simulink model "simulation2"  (R2021a)
settings: Solver=FixedStepAuto  StartTime=0.0  StopTime=10.0  RelTol=1e-3
values from neighbouring files (symbols this model uses):
  g = 9.8    [invertedp.m]
  K = [-35 -34 -150 -34]    [invertedp.m]
undefined symbols (not defined in the file or in its folder): a, F_v, iM_d, iner, iner_l, K_d, K_p, o_r, pi_l, pi_m, q_i, Tc
settings Model: Creator=jonathanbopp  LastModifiedBy=jonathanbopp

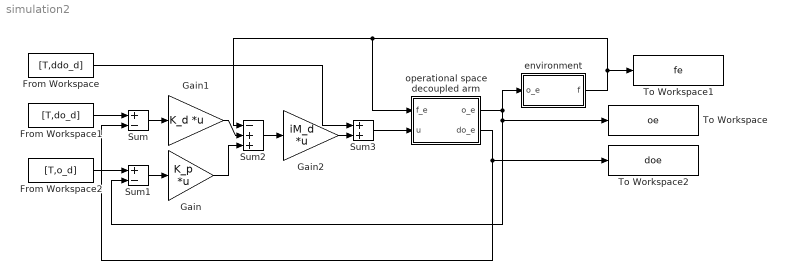
== system simulation2 ==
  From Workspace : FromWorkspace  VariableName=[T,ddo_d]  SampleTime=Tc
  From Workspace1 : FromWorkspace  VariableName=[T,do_d]  SampleTime=Tc
  From Workspace2 : FromWorkspace  VariableName=[T,o_d]  SampleTime=Tc
  Gain : Gain  Gain=K_p  Multiplication=Matrix(K*u)
  Gain1 : Gain  Gain=K_d  Multiplication=Matrix(K*u)
  Gain2 : Gain  Gain=iM_d  Multiplication=Matrix(K*u)
  Sum : Sum  Inputs=+-
  Sum1 : Sum  Inputs=+-
  Sum2 : Sum  Inputs=-||+||+
  Sum3 : Sum
  To Workspace : ToWorkspace  VariableName=oe  SaveFormat=Timeseries  SampleTime=-1
  To Workspace1 : ToWorkspace  VariableName=fe  SaveFormat=Timeseries  SampleTime=-1
  To Workspace2 : ToWorkspace  VariableName=doe  SaveFormat=Timeseries  SampleTime=-1
  environment : Subsystem
      mask Display: disp('K(o_e-o_r)')
  operational space decoupled arm : Subsystem
      mask Display: disp('u = ddo_e')
  wires:
  operational space decoupled arm/1(o_e) -> To Workspace/1, Sum1/2, environment/1(o_e)
  Sum3/1 -> operational space decoupled arm/2(u)
  From Workspace2/1 -> Sum1/1
  Sum1/1 -> Gain/1
  Gain/1 -> Sum2/3
  Gain1/1 -> Sum2/2
  Sum/1 -> Gain1/1
  From Workspace1/1 -> Sum/1
  Sum2/1 -> Gain2/1
  Gain2/1 -> Sum3/2
  From Workspace/1 -> Sum3/1
  environment/1(f) -> To Workspace1/1, operational space decoupled arm/1(f_e), Sum2/1
  operational space decoupled arm/2(do_e) -> To Workspace2/1, Sum/2

== system simulation2/environment ==
  o_e : Inport
  Matrix gain. : StateSpace  A=[]  B=[]  C=[]  D=K  InitialCondition=0  mask(Matrix gain){K=K}
      mask prompts: K "Gain matrix:"
      mask help: Matrix Gain.
      mask Help: Multiplies input vector by entered matrix to produce output vector (y=Au).
      mask Display: disp('K')
  Sum1 : Sum  Inputs=+-  InputSameDT=on  SaturateOnIntegerOverflow=on  OutDataTypeStr=Inherit: Same as first input
  xo : Constant  Value=o_r  SampleTime=-1
  f : Outport  InitialOutput=0
  wires:
  o_e/1 -> Sum1/1
  Matrix gain./1 -> f/1
  Sum1/1 -> Matrix gain./1
  xo/1 -> Sum1/2

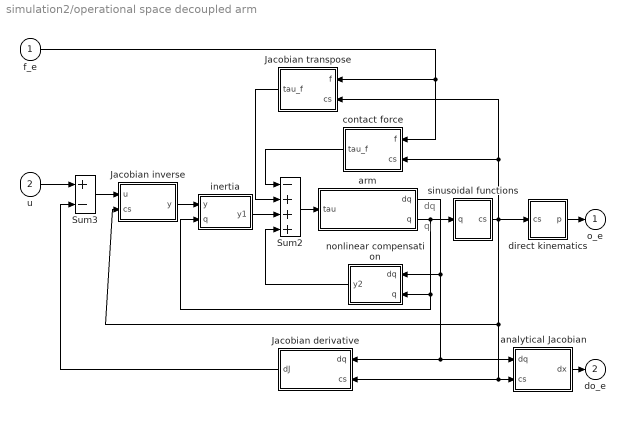
== system simulation2/operational space decoupled arm ==
  note: dq
  note: q
  f_e : Inport
  u : Inport  Port=2
  Jacobian derivative : Subsystem
      mask Display: disp('dJ_a(q,dq)')
  Jacobian inverse : Subsystem
      mask Display: disp('inv(J_a(q))')
  Jacobian transpose : Subsystem
      mask Display: disp('tr(J_a(q))')
  Sum2 : Sum  Inputs=-+++  InputSameDT=on  SaturateOnIntegerOverflow=on  OutDataTypeStr=Inherit: Same as first input
  Sum3 : Sum  Inputs=+-  InputSameDT=on  SaturateOnIntegerOverflow=on  OutDataTypeStr=Inherit: Same as first input
  analytical Jacobian : Subsystem
      mask Display: disp('J_a(q)')
  arm : Subsystem
      mask Display: disp('inv(B(q))(tau-tau'')')
  contact force : Subsystem
      mask Display: disp('tr(J_a(q))f')
  direct kinematics : Subsystem
      mask Display: disp('k(q)')
  inertia : Subsystem
      mask Display: disp('B(q)')
  nonlinear compensation : Subsystem
      mask Display: disp('n(q,dq)')
  sinusoidal functions : Subsystem
      mask Display: disp('cs(q)')
  o_e : Outport  InitialOutput=0
  do_e : Outport  Port=2  InitialOutput=0
  wires:
  f_e/1 -> contact force/1(f), Jacobian transpose/1(f)
  Jacobian transpose/1(tau_f) -> Sum2/2
  inertia/1(y1) -> Sum2/3
  nonlinear compensation/1(y2) -> Sum2/4
  Jacobian derivative/1(dJ) -> Sum3/2
  u/1 -> Sum3/1
  sinusoidal functions/1(cs) -> Jacobian inverse/2(cs), Jacobian derivative/2(cs), analytical Jacobian/2(cs), Jacobian transpose/2(cs), contact force/2(cs), direct kinematics/1(cs)
  contact force/1(tau_f) -> Sum2/1
  arm/2("q ") -> inertia/2(q), nonlinear compensation/2(q), sinusoidal functions/1(q)
  Sum3/1 -> Jacobian inverse/1(u)
  analytical Jacobian/1(dx) -> do_e/1
  direct kinematics/1(p) -> o_e/1
  arm/1(dq) -> nonlinear compensation/1(dq), Jacobian derivative/1(dq), analytical Jacobian/1(dq)
  Sum2/1 -> arm/1(tau)
  Jacobian inverse/1(y) -> inertia/1(y)

== system simulation2/operational space decoupled arm/Jacobian derivative ==
  dq : Inport
  cs : Inport  Port=2
  MATLAB Fcn : MATLABFcn  MATLABFcn=dJ_a  OutputDimensions=2  SampleTime=Tc
      mask Display: disp('dJ_a(q,dq)dq')
  Mux : Mux  Inputs=[2,4]
  dJ : Outport  InitialOutput=0
  wires:
  MATLAB Fcn/1 -> dJ/1
  Mux/1 -> MATLAB Fcn/1
  cs/1 -> Mux/2
  dq/1 -> Mux/1

== system simulation2/operational space decoupled arm/Jacobian inverse ==
  u : Inport
  cs : Inport  Port=2
  MATLAB Fcn : MATLABFcn  MATLABFcn=invJ_a  OutputDimensions=2  SampleTime=Tc
      mask Display: disp('inv(J_a(q))')
  Mux : Mux  Inputs=[2,4]
  y : Outport  InitialOutput=0
  wires:
  u/1 -> Mux/1
  cs/1 -> Mux/2
  Mux/1 -> MATLAB Fcn/1
  MATLAB Fcn/1 -> y/1

== system simulation2/operational space decoupled arm/Jacobian transpose ==
  f : Inport
  cs : Inport  Port=2
  MATLAB Fcn : MATLABFcn  MATLABFcn=trJ_a  OutputDimensions=2  SampleTime=Tc
      mask Display: disp('J''_a(q)f')
  Mux : Mux  Inputs=[2,4]
  tau_f : Outport  InitialOutput=0
  wires:
  cs/1 -> Mux/2
  f/1 -> Mux/1
  Mux/1 -> MATLAB Fcn/1
  MATLAB Fcn/1 -> tau_f/1

== system simulation2/operational space decoupled arm/analytical Jacobian ==
  dq : Inport
  cs : Inport  Port=2
  MATLAB Fcn : MATLABFcn  MATLABFcn=J_adq  OutputDimensions=2
      mask Display: disp('J_a(q)dq')
  Mux : Mux  Inputs=[2,4]
  dx : Outport  InitialOutput=0
  wires:
  cs/1 -> Mux/2
  MATLAB Fcn/1 -> dx/1
  Mux/1 -> MATLAB Fcn/1
  dq/1 -> Mux/1

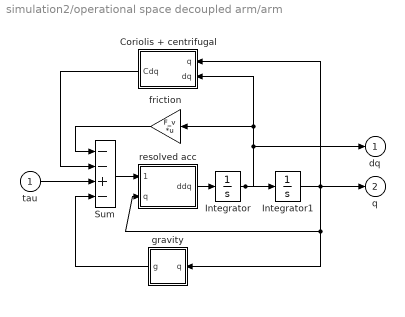
== system simulation2/operational space decoupled arm/arm ==
  tau : Inport
  Coriolis + centrifugal : Subsystem
      mask Display: disp('C(q,dq)dq')
  Integrator : Integrator  InitialCondition=[0 0]  ZeroCross=off
  Integrator1 : Integrator  InitialCondition=q_i  ZeroCross=off
  Sum : Sum  Inputs=--+-  InputSameDT=on  SaturateOnIntegerOverflow=on  OutDataTypeStr=Inherit: Same as first input
  friction : Gain  Gain=F_v  Multiplication=Matrix(K*u)  SaturateOnIntegerOverflow=on  OutDataTypeStr=Inherit: Same as input  ParamDataTypeStr=Inherit: Same as input
      mask Display: disp('F_v')
  gravity : Subsystem
      mask Display: disp('g(q)')
  resolved acc : Subsystem
      mask Display: disp('inv(B(q))')
  dq : Outport  InitialOutput=0
  "q " : Outport  Port=2  InitialOutput=0
  wires:
  gravity/1(g) -> Sum/4
  friction/1 -> Sum/1
  Sum/1 -> resolved acc/1(tau-tau')
  Integrator/1 -> friction/1, Coriolis + centrifugal/2(dq), dq/1, Integrator1/1
  resolved acc/1(ddq) -> Integrator/1
  Integrator1/1 -> "q "/1, gravity/1(q), resolved acc/2(q), Coriolis + centrifugal/1(q)
  tau/1 -> Sum/3
  Coriolis + centrifugal/1(Cdq) -> Sum/2

== system simulation2/operational space decoupled arm/contact force ==
  f : Inport
  cs : Inport  Port=2
  MATLAB Fcn : MATLABFcn  MATLABFcn=trJ_a  OutputDimensions=2
      mask Display: disp('J''_a(q)f')
  Mux : Mux  Inputs=[2,4]
  tau_f : Outport  InitialOutput=0
  wires:
  MATLAB Fcn/1 -> tau_f/1
  Mux/1 -> MATLAB Fcn/1
  cs/1 -> Mux/2
  f/1 -> Mux/1

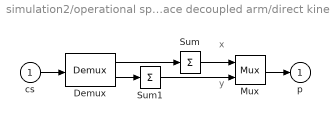
== system simulation2/operational space decoupled arm/direct kinematics ==
  note: y
  note: x
  cs : Inport
  Demux : Demux  Outputs=[2,2]
      settings: DisplayOption=none
  Mux : Mux  Inputs=2
  Sum : Sum  Inputs=+  InputSameDT=on  SaturateOnIntegerOverflow=on  OutDataTypeStr=Inherit: Same as first input
  Sum1 : Sum  Inputs=+  InputSameDT=on  SaturateOnIntegerOverflow=on  OutDataTypeStr=Inherit: Same as first input
  p : Outport  InitialOutput=0
  wires:
  Mux/1 -> p/1
  cs/1 -> Demux/1
  Demux/1 -> Sum/1
  Demux/2 -> Sum1/1
  Sum/1 -> Mux/1
  Sum1/1 -> Mux/2

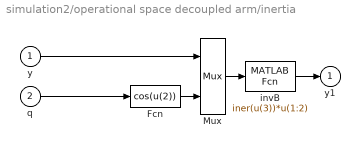
== system simulation2/operational space decoupled arm/inertia ==
  y : Inport
  q : Inport  Port=2
  Fcn : Fcn  Expr=cos(u(2))  SampleTime=Tc
  Mux : Mux  Inputs=[2,1]
  "invB " : MATLABFcn  MATLABFcn=iner(u(3))*u(1:2)  OutputDimensions=2  SampleTime=Tc
      mask Display: disp('B(q)y')
  y1 : Outport  InitialOutput=0
  wires:
  y/1 -> Mux/1
  q/1 -> Fcn/1
  Mux/1 -> "invB "/1
  "invB "/1 -> y1/1
  Fcn/1 -> Mux/2

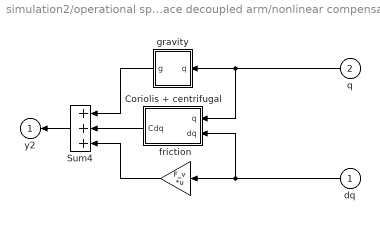
== system simulation2/operational space decoupled arm/nonlinear compensation ==
  dq : Inport
  q : Inport  Port=2
  Coriolis + centrifugal : Subsystem
      mask Display: disp('C(q,dq)dq')
  Sum4 : Sum  Inputs=+++  InputSameDT=on  SaturateOnIntegerOverflow=on  OutDataTypeStr=Inherit: Same as first input
  friction : Gain  Gain=F_v  Multiplication=Matrix(K*u)  SaturateOnIntegerOverflow=on  SampleTime=Tc  OutDataTypeStr=Inherit: Same as input  ParamDataTypeStr=Inherit: Same as input
      mask Display: disp('F_v')
  gravity : Subsystem
      mask Display: disp('g(q)')
  y2 : Outport  InitialOutput=0
  wires:
  Coriolis + centrifugal/1(Cdq) -> Sum4/2
  dq/1 -> friction/1, Coriolis + centrifugal/2(dq)
  q/1 -> Coriolis + centrifugal/1(q), gravity/1(q)
  friction/1 -> Sum4/3
  Sum4/1 -> y2/1
  gravity/1(g) -> Sum4/1

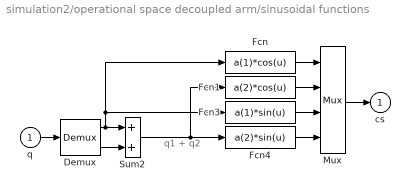
== system simulation2/operational space decoupled arm/sinusoidal functions ==
  note: q1 + q2
  q : Inport
  Demux : Demux  Outputs=2
      settings: DisplayOption=none
  Fcn : Fcn  Expr=a(1)*cos(u)
  Fcn1 : Fcn  Expr=a(2)*cos(u)
  Fcn3 : Fcn  Expr=a(1)*sin(u)
  Fcn4 : Fcn  Expr=a(2)*sin(u)
  Mux : Mux
  Sum2 : Sum  InputSameDT=on  SaturateOnIntegerOverflow=on  OutDataTypeStr=Inherit: Same as first input
  cs : Outport  InitialOutput=0
  wires:
  Fcn/1 -> Mux/1
  Mux/1 -> cs/1
  Demux/1 -> Sum2/1, Fcn3/1, Fcn/1
  Demux/2 -> Sum2/2
  Sum2/1 -> Fcn4/1, Fcn1/1
  Fcn1/1 -> Mux/2
  Fcn3/1 -> Mux/3
  Fcn4/1 -> Mux/4
  q/1 -> Demux/1

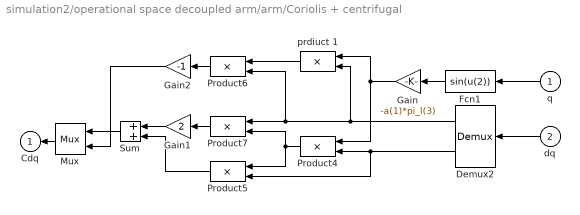
== system simulation2/operational space decoupled arm/arm/Coriolis + centrifugal ==
  q : Inport
  dq : Inport  Port=2
  Demux2 : Demux  Outputs=2
      settings: DisplayOption=none
  Fcn1 : Fcn  Expr=sin(u(2))
  Gain : Gain  Gain=-a(1)*pi_l(3)  SaturateOnIntegerOverflow=on  OutDataTypeStr=Inherit: Same as input  ParamDataTypeStr=Inherit: Same as input
      mask Display: disp('k_3')
  Gain1 : Gain  Gain=2  SaturateOnIntegerOverflow=on  OutDataTypeStr=Inherit: Same as input  ParamDataTypeStr=Inherit: Same as input
  Gain2 : Gain  Gain=-1  SaturateOnIntegerOverflow=on  OutDataTypeStr=Inherit: Same as input  ParamDataTypeStr=Inherit: Same as input
  Mux : Mux  Inputs=2
  Product{4..7} (4 alike) : Product  InputSameDT=on  RndMeth=Zero  SaturateOnIntegerOverflow=on  OutDataTypeStr=Inherit: Same as first input
  Sum : Sum  InputSameDT=on  SaturateOnIntegerOverflow=on  OutDataTypeStr=Inherit: Same as first input
  prdiuct 1 : Product  InputSameDT=on  RndMeth=Zero  SaturateOnIntegerOverflow=on  OutDataTypeStr=Inherit: Same as first input
  Cdq : Outport  InitialOutput=0
  wires:
  Product4/1 -> Product7/2, Product5/1
  q/1 -> Fcn1/1
  Fcn1/1 -> Gain/1
  Gain/1 -> Product4/1, prdiuct 1/1
  prdiuct 1/1 -> Product6/1
  Demux2/2 -> Product5/2, Product4/2
  Demux2/1 -> Product7/1, Product6/2, prdiuct 1/2
  Product7/1 -> Gain1/1
  Gain1/1 -> Sum/1
  Product5/1 -> Sum/2
  Sum/1 -> Mux/1
  Mux/1 -> Cdq/1
  Product6/1 -> Gain2/1
  Gain2/1 -> Mux/2
  dq/1 -> Demux2/1

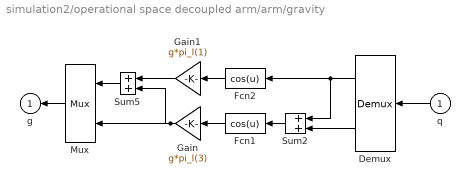
== system simulation2/operational space decoupled arm/arm/gravity ==
  q : Inport
  Demux : Demux  Outputs=2
      settings: DisplayOption=none
  Fcn1 : Fcn  Expr=cos(u)
  Fcn2 : Fcn  Expr=cos(u)
  Gain : Gain  Gain=g*pi_l(3)  SaturateOnIntegerOverflow=on  OutDataTypeStr=Inherit: Same as input  ParamDataTypeStr=Inherit: Same as input
      mask Display: disp('k_2')
  Gain1 : Gain  Gain=g*pi_l(1)  SaturateOnIntegerOverflow=on  OutDataTypeStr=Inherit: Same as input  ParamDataTypeStr=Inherit: Same as input
      mask Display: disp('k_1')
  Mux : Mux  Inputs=2
  Sum2 : Sum  InputSameDT=on  SaturateOnIntegerOverflow=on  OutDataTypeStr=Inherit: Same as first input
  Sum5 : Sum  InputSameDT=on  SaturateOnIntegerOverflow=on  OutDataTypeStr=Inherit: Same as first input
  g : Outport  InitialOutput=0
  wires:
  Mux/1 -> g/1
  Gain/1 -> Mux/2, Sum5/2
  Sum5/1 -> Mux/1
  Gain1/1 -> Sum5/1
  Demux/1 -> Sum2/1, Fcn2/1
  Fcn2/1 -> Gain1/1
  Fcn1/1 -> Gain/1
  Sum2/1 -> Fcn1/1
  Demux/2 -> Sum2/2
  q/1 -> Demux/1

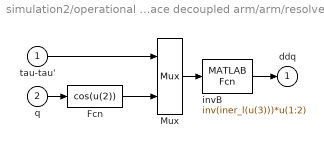
== system simulation2/operational space decoupled arm/arm/resolved acc ==
  tau-tau' : Inport
  q : Inport  Port=2
  Fcn : Fcn  Expr=cos(u(2))
  Mux : Mux  Inputs=[2,1]
  "invB " : MATLABFcn  MATLABFcn=inv(iner_l(u(3)))*u(1:2)  OutputDimensions=2
      mask Display: disp('inv(B(q))')
  ddq : Outport  InitialOutput=0
  wires:
  Mux/1 -> "invB "/1
  tau-tau'/1 -> Mux/1
  "invB "/1 -> ddq/1
  q/1 -> Fcn/1
  Fcn/1 -> Mux/2

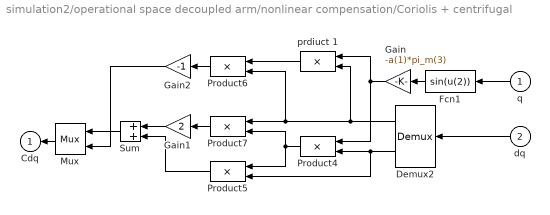
== system simulation2/operational space decoupled arm/nonlinear compensation/Coriolis + centrifugal ==
  q : Inport
  dq : Inport  Port=2
  Demux2 : Demux  Outputs=2
      settings: DisplayOption=none
  Fcn1 : Fcn  Expr=sin(u(2))  SampleTime=Tc
  Gain : Gain  Gain=-a(1)*pi_m(3)  SaturateOnIntegerOverflow=on  OutDataTypeStr=Inherit: Same as input  ParamDataTypeStr=Inherit: Same as input
      mask Display: disp('k_3')
  Gain1 : Gain  Gain=2  SaturateOnIntegerOverflow=on  OutDataTypeStr=Inherit: Same as input  ParamDataTypeStr=Inherit: Same as input
  Gain2 : Gain  Gain=-1  SaturateOnIntegerOverflow=on  OutDataTypeStr=Inherit: Same as input  ParamDataTypeStr=Inherit: Same as input
  Mux : Mux  Inputs=2
  Product{4..7} (4 alike) : Product  InputSameDT=on  RndMeth=Zero  SaturateOnIntegerOverflow=on  SampleTime=Tc  OutDataTypeStr=Inherit: Same as first input
  Sum : Sum  InputSameDT=on  SaturateOnIntegerOverflow=on  OutDataTypeStr=Inherit: Same as first input
  prdiuct 1 : Product  InputSameDT=on  RndMeth=Zero  SaturateOnIntegerOverflow=on  SampleTime=Tc  OutDataTypeStr=Inherit: Same as first input
  Cdq : Outport  InitialOutput=0
  wires:
  Demux2/2 -> Product5/2, Product4/2
  dq/1 -> Demux2/1
  q/1 -> Fcn1/1
  Gain2/1 -> Mux/2
  Product6/1 -> Gain2/1
  Mux/1 -> Cdq/1
  Sum/1 -> Mux/1
  Product5/1 -> Sum/2
  Gain1/1 -> Sum/1
  Product7/1 -> Gain1/1
  prdiuct 1/1 -> Product6/1
  Gain/1 -> Product4/1, prdiuct 1/1
  Fcn1/1 -> Gain/1
  Demux2/1 -> Product7/1, Product6/2, prdiuct 1/2
  Product4/1 -> Product7/2, Product5/1

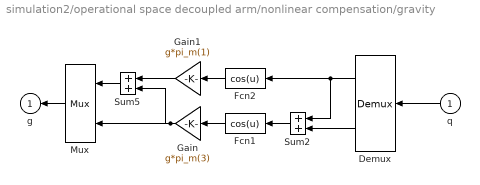
== system simulation2/operational space decoupled arm/nonlinear compensation/gravity ==
  q : Inport
  Demux : Demux  Outputs=2
      settings: DisplayOption=none
  Fcn1 : Fcn  Expr=cos(u)  SampleTime=Tc
  Fcn2 : Fcn  Expr=cos(u)  SampleTime=Tc
  Gain : Gain  Gain=g*pi_m(3)  SaturateOnIntegerOverflow=on  OutDataTypeStr=Inherit: Same as input  ParamDataTypeStr=Inherit: Same as input
      mask Display: disp('k_2')
  Gain1 : Gain  Gain=g*pi_m(1)  SaturateOnIntegerOverflow=on  OutDataTypeStr=Inherit: Same as input  ParamDataTypeStr=Inherit: Same as input
      mask Display: disp('k_1')
  Mux : Mux  Inputs=2
  Sum2 : Sum  InputSameDT=on  SaturateOnIntegerOverflow=on  SampleTime=Tc  OutDataTypeStr=Inherit: Same as first input
  Sum5 : Sum  InputSameDT=on  SaturateOnIntegerOverflow=on  OutDataTypeStr=Inherit: Same as first input
  g : Outport  InitialOutput=0
  wires:
  Mux/1 -> g/1
  Gain/1 -> Sum5/2, Mux/2
  Sum5/1 -> Mux/1
  Gain1/1 -> Sum5/1
  Demux/1 -> Sum2/1, Fcn2/1
  Fcn2/1 -> Gain1/1
  Fcn1/1 -> Gain/1
  Sum2/1 -> Fcn1/1
  Demux/2 -> Sum2/2
  q/1 -> Demux/1
